simulink model "CPower_LKA"  (R2018a)
settings: Solver=VariableStepAuto  StartTime=0.0  StopTime=10.0  RelTol=1e-3
libraries: vehdynlibsteering x1, dspvision x1
settings Model: Creator=ciara  LastModifiedBy=ciara

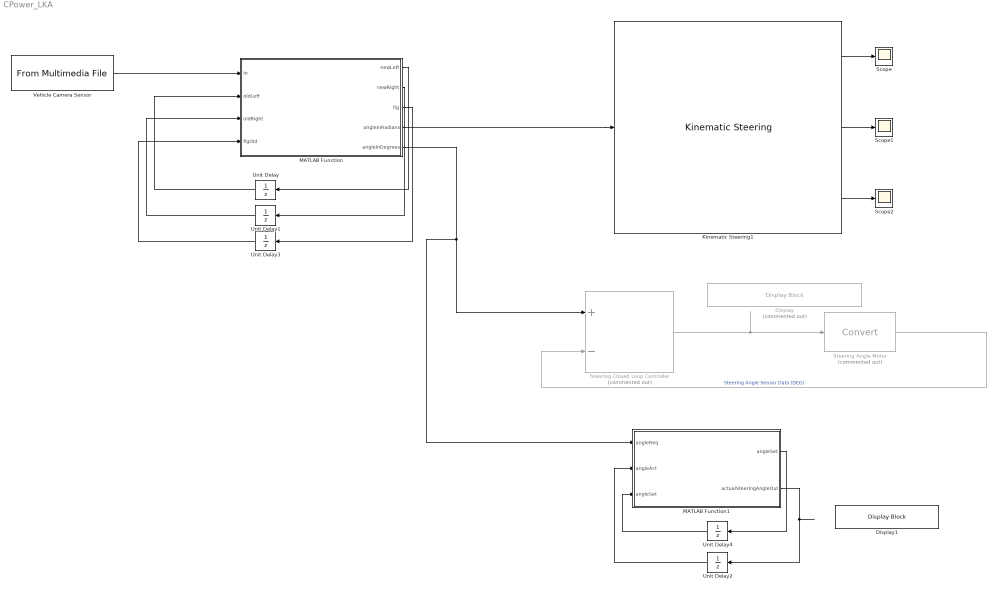
== system CPower_LKA ==
  Display : DisplayBlock  Commented=on  WebBlockId=23  LabelPosition=Hide
  Display1 : DisplayBlock  WebBlockId=32  LabelPosition=Hide
  Kinematic Steering1 : vehdynlibsteering/Kinematic Steering  StrgType=Parallel  StrgRatioType=Constant  Loc=Front  NrmlFctr=0.01  TrckWdth=1  WhlBase=1.524  Db=0  StrgRng=1.25*pi  StrgAngBpts="[-6.2832   -5.0265   -3.7699   -2.5133   -1.2566         0    1.2566    2.5133    3.7699    5.0265    6.2832]"  StrgRatioTbl=|  StrgRatio=100  StrgArmLngth=0.1  RckCsLngth=0.5  TieRodLngth=0.248  D=0.2  PnnRadius=0.0057  PnnRadiusTbl="[0.0055    0.0055    0.0056    0.0057    0.0058    0.0057    0.0057    0.0057    0.0056    0.0055    0.0055]"  RodLngth=0.1  ParaArmLngth=0.9  aMode=2
      | [13.5000   13.3750   13.2500   13.1250   13.0000   13.0000   13.0000   13.1250   13.2500   13.3750   13.5000
      | ]
      settings: SourceProductName=Vehicle Dynamics Blockset
  MATLAB Function : MATLAB Function  TreatAsAtomicUnit=on
  MATLAB Function1 : MATLAB Function  TreatAsAtomicUnit=on
  Scope : Scope
  Scope1 : Scope
  Scope2 : Scope
  Steering Angle Motor : DataTypeConversion  Commented=on
  Steering Closed Loop Controller : Sum  Commented=on  Inputs=+-
  Unit Delay{,1..4} (5 alike) : UnitDelay  SampleTime=-1
  Vehicle Camera Sensor : dspvision/From Multimedia File  inputFilename=C:\Users\ciara\OneDrive - Waterford Institute of Technology\Applied_computing\4th_year\Semester_1\ADAS\CPower_LKA\LKA_input.mp4  loop=on  numPlays=inf  outputStreams=Video only  videoDataType=single  audioDataType=int16  inheritSampleTime=on  userDefinedSampleTime=1/30  noAudioOutput=off  isIntensityVideo=off  fourcc=RGB  colorVideoFormat=One multidimensional signal  outputEOF=off  dataOrg=Column-major  audioFrameSize=1024  computeAudioFrameSize=off  outSamplingMode=Sample based
      settings: SourceProductBaseCode=VP
  wires:
  MATLAB Function/1(newLeft) -> Unit Delay/1
  Unit Delay/1 -> MATLAB Function/2(oldLeft)
  MATLAB Function/2(newRight) -> Unit Delay1/1
  Unit Delay1/1 -> MATLAB Function/3(oldRight)
  MATLAB Function/3(fig) -> Unit Delay3/1
  Unit Delay3/1 -> MATLAB Function/4(figOld)
  MATLAB Function/4(angleInRadians) -> Kinematic Steering1/1
  Kinematic Steering1/1 -> Scope/1
  Kinematic Steering1/2 -> Scope1/1
  Kinematic Steering1/3 -> Scope2/1
  Vehicle Camera Sensor/1 -> MATLAB Function/1(In)
  Steering Closed Loop Controller/1 -> Steering Angle Motor/1
  MATLAB Function/5(angleInDegrees) -> MATLAB Function1/1(angleReq), Steering Closed Loop Controller/1
  Steering Angle Motor/1 -> Steering Closed Loop Controller/2  "Steering Angle Sensor Data (DEG)"
  MATLAB Function1/2(actualSteeringAngleOut) -> Unit Delay2/1
  Unit Delay2/1 -> MATLAB Function1/2(angleAct)
  MATLAB Function1/1(angleSet) -> Unit Delay4/1
  Unit Delay4/1 -> MATLAB Function1/3("angleSet ")

== matlab function CPower_LKA/MATLAB Function1 ==
  data: angleSet output; angleReq input; actualSteeringAngleOut output; angleAct input; angleSet input
function [angleSet,actualSteeringAngleOut] = steeringAngleController(angleReq, angleAct,angleSet)

if not(angleSet)
  angleAct = 90; %% assume 90 starting point
end

if(angleReq>angleAct)
    actualSteeringAngleOut = angleAct+1;
    angleSet =1;
    
elseif (angleReq<angleAct)
    actualSteeringAngleOut = angleAct-1;
    angleSet =1;
else
    actualSteeringAngleOut = angleAct;
    angleSet =1;
end

== matlab function CPower_LKA/MATLAB Function ==
  data: In input; newLeft output; newRight output; oldLeft input; oldRight input; figOld input; fig output; angleInRadians output; angleInDegrees output
function [newLeft, newRight, fig, angleInRadians, angleInDegrees] =  lane_keep_assist(In, oldLeft, oldRight, figOld)

fig = zeros(1,3);
newLeft = zeros(2,2);
newRight = zeros(2,2);
angleInRadians=0;
angleInDegrees=90;

coder.extrinsic('imshow');
coder.extrinsic('polyxpoly');
coder.extrinsic('num2str');
coder.extrinsic('strcat');
coder.extrinsic('deg2rad');

if isempty(figOld)
    fig = figure;
else 
    fig = figOld;
    cla(fig);
end 

[rows, columns, z1] = size(In);
height = rows;
width = columns;
I = imcrop(In,[width*.3 height*.78 width*.4 height*.2]);

IG=rgb2gray(I);

bw = imbinarize(IG, 0.85);

BWCL=bwmorph(bw,'clean');

BWSKEL=bwmorph(BWCL,'skel',Inf);

BW = edge(BWSKEL,'roberts');

[H,T,R] = hough(BW, 'Theta',-75:75);

%{ 
% Display Hough transform output
imshow(imadjust(rescale(H)),'XData',T,'YData',R,...
      'InitialMagnification','fit');
title('Hough transform');
xlabel('\theta'), ylabel('\rho');
axis on, axis normal, hold on;
colormap(gca,hot);
%}

P  = houghpeaks(H,100,'threshold',ceil(0.3*max(H(:))));
x = T(P(:,2)); y = R(P(:,1));
%Plot Peaks on Hough Transform Graph
% plot(x,y,'s','color','white');


lines = houghlines(BW,T,R,P,'FillGap',10,'MinLength',0.01);
imshow(In), hold on
max_len1 = 0;
xy_left=[0 0;0 0];
max_len2 = 0;
xy_right=[0 0; 0 0];
for k = 1:length(lines)
    
   xy = [lines(k).point1; lines(k).point2];
   % Get the equation of the line
   x1 = xy(1,1)+width*.3;
   y1 = xy(1,2)+height*.78;
   x2 = xy(2,1)+width*.3;
   y2 = xy(2,2)+height*.78;
   slope = (y2-y1)/(x2-x1);
   xLeft = 1;
   yLeft = slope * (xLeft - x1) + y1;
   xRight = columns;
   yRight = slope * (xRight - x1) + y1; 
    xy(1,1) = xLeft;
    xy(1,2) = yLeft;
    xy(2,1)= xRight;
    xy(2,2) = yRight;
 
   % Determine the length of the line segment
   len = norm(lines(k).point1 - lines(k).point2);
   
   if ( slope < 0 && len > max_len1 )
      max_len1 = len;
      xy_left = xy;
   elseif ( slope > 0 && len > max_len2 )
           max_len2 = len;
           xy_right = xy;
   end   
end

if(isequal(xy_left,[0 0;0 0]))
    xy_left=oldLeft;
elseif(not(isequal(oldLeft,[0 0;0 0])))
    xy_left = (xy_left + oldLeft) /2;
end

if(isequal(xy_right,[0 0;0 0]))
    xy_right=oldRight;
elseif(not(isequal(oldRight,[0 0;0 0])))
    xy_right = (xy_right + oldRight) /2;
end
plot(xy_left(:,1),xy_left(:,2),'LineWidth',3,'Color','cyan');
xLeftStart = interp1(xy_left(:,2),xy_left(:,1), height, 'linear');
xRightStart = interp1(xy_right(:,2),xy_right(:,1), height, 'linear');

if(not(xLeftStart < xRightStart))
    xy_left = oldLeft;
    xy_right = oldRight;
    xLeftStart = interp1(xy_left(:,2),xy_left(:,1), height, 'linear');
    xRightStart = interp1(xy_right(:,2),xy_right(:,1), height, 'linear');
end

[intersect_x, intersect_y] = polyxpoly(xy_left(:,1), xy_left(:,2),xy_right(:,1),xy_right(:,2), 'unique');

plot(xy_left(:,1),xy_left(:,2),'LineWidth',3,'Color','cyan');
plot(xy_right(:,1),xy_right(:,2),'LineWidth',3,'Color','blue');

plot(intersect_x, intersect_y,'x', 'LineWidth',2,'Color','red');
plot(width/2, height,'x', 'LineWidth',2,'Color','green');

plot(xLeftStart, height,'x', 'LineWidth',2,'Color','white');
plot(xRightStart, height,'x', 'LineWidth',2,'Color','white');

centerX = xLeftStart+((xRightStart-xLeftStart)/2);
plot(centerX, height,'x', 'LineWidth',2,'Color','yellow');

intersect_y_num =0;
intersect_y_num = intersect_y;
intersect_x_num =0;
intersect_x_num = intersect_x;


yRefPoint = height- (height-intersect_y_num)/2;
plot([centerX intersect_x_num],[height intersect_y_num],'LineWidth',2,'Color','yellow');
xRefPoint = interp1([height intersect_y_num],[centerX intersect_x_num], yRefPoint, 'linear');
plot(xRefPoint, yRefPoint,'x', 'LineWidth',2,'Color','magenta');

angleInDegrees = atan2d(yRefPoint-height, xRefPoint-width/2);
if (angleInDegrees<0)
    angleInDegrees=angleInDegrees*-1;
end

steeringDegAngle = 0;
steeringDegAngle = angleInDegrees;
steerString =  num2str(steeringDegAngle,'%.0f');

if (steeringDegAngle<89.5)
    text(0.25, 30, strcat('Turn Right to ',{' '},steerString,char(176)), 'FontSize',24,'Color','r');
elseif(steeringDegAngle>90.5)
    text(0.25, 30, strcat('Turn Left to ',{' '},steerString,char(176)),'FontSize',24,'Color','r');
else 
    text(0.25, 30, strcat('Continue : ',{' '},steerString,char(176)),'FontSize',24,'Color','r');
end

newLeft =  [xy_left(1,1) xy_left(1,2); xy_left(2,1) xy_left(2,2)];
newRight = [xy_right(1,1) xy_right(1,2); xy_right(2,1) xy_right(2,2)];

angleInRadians = deg2rad(angleInDegrees-90) ;
